simulink model "problem2"  (R2020b)
settings: Solver=VariableStepAuto  StartTime=0.0  StopTime=10.0  RelTol=1e-3
model workspace (MAT data in the model file):
  K1 = Simulink.Parameter
  K1.Value = 1
  K1.DataType = 'auto'
  K1.Dimensions = [1 1]
  K2 = Simulink.Parameter
  K2.Value = 1
  K2.DataType = 'auto'
  K2.Dimensions = [1 1]
  M2 = Simulink.Parameter
  M2.Value = 1
  M2.DataType = 'auto'
  M2.Dimensions = [1 1]
undefined symbols (not defined in the file): b, M1
settings Model: Creator=admin  LastModifiedBy=admin

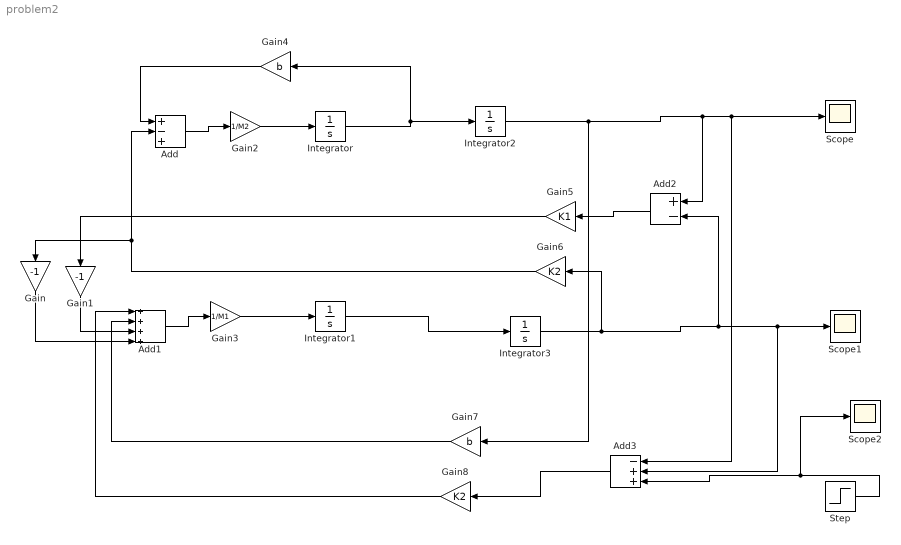
== system problem2 ==
  Add : Sum  Inputs=+-+
  Add1 : Sum  Inputs=++++
  Add2 : Sum  Inputs=+-
  Add3 : Sum  Inputs=-++
  Gain : Gain  Gain=-1
  Gain1 : Gain  Gain=-1
  Gain2 : Gain  Gain=1/M2
  Gain3 : Gain  Gain=1/M1
  Gain4 : Gain  Gain=b
  Gain5 : Gain  Gain=K1
  Gain6 : Gain  Gain=K2
  Gain7 : Gain  Gain=b
  Gain8 : Gain  Gain=K2
  Integrator{,1..3} (4 alike) : Integrator
  Scope : Scope
  Scope1 : Scope
  Scope2 : Scope
  Step : Step  SampleTime=0
  wires:
  Integrator2/1 -> Add2/1, Add3/1, Scope/1, Gain7/1
  Integrator/1 -> Gain4/1, Integrator2/1
  Gain4/1 -> Add/1
  Gain5/1 -> Gain1/1
  Add2/1 -> Gain5/1
  Integrator3/1 -> Gain6/1, Add2/2, Add3/2, Scope1/1
  Integrator1/1 -> Integrator3/1
  Gain3/1 -> Integrator1/1
  Add1/1 -> Gain3/1
  Gain1/1 -> Add1/3
  Gain/1 -> Add1/4
  Gain6/1 -> Gain/1, Add/2
  Step/1 -> Scope2/1, Add3/3
  Gain7/1 -> Add1/2
  Gain8/1 -> Add1/1
  Add3/1 -> Gain8/1
  Gain2/1 -> Integrator/1
  Add/1 -> Gain2/1
